simulink model "dragEffects"  (R2016b)
settings: Solver=ode113  StartTime=0.0  StopTime=.5*86400  MaxStep=60  RelTol=1e-6  AbsTol=1e-9
values from neighbouring files (symbols this model uses):
  i = .7854    (= 0.7854)    [PS8.m]
  rINT = [6613.137; 0; 0]    [PS8.m]
  vINT = [0; 7.763631; 0]    [PS8.m]
undefined symbols (not defined in the file or in its folder): AoP, RAAN
settings Model: Creator=rushalrege  LastModifiedBy=rushalrege

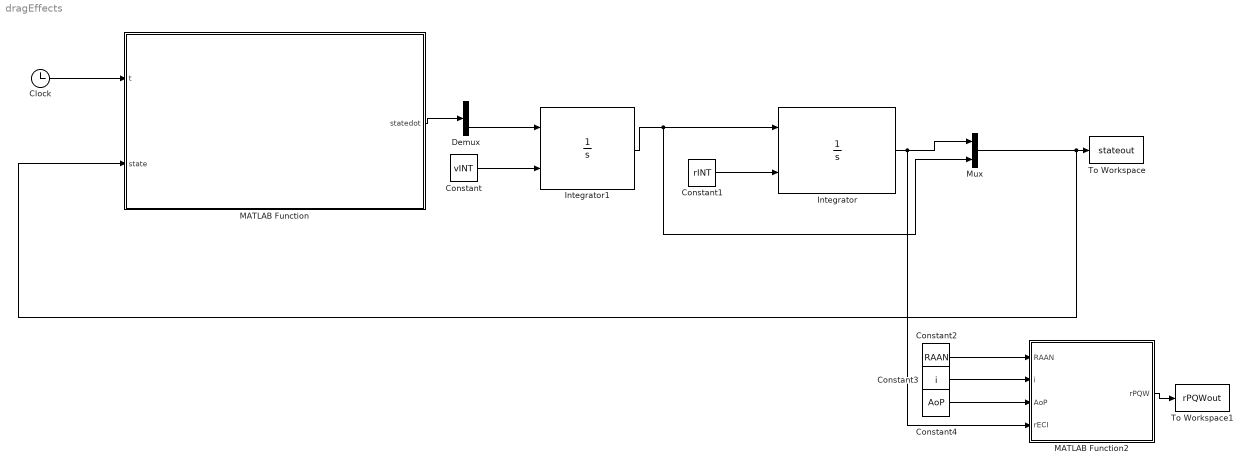
== system dragEffects ==
  Clock : Clock
  Constant : Constant  Value=vINT
  Constant1 : Constant  Value=rINT
  Constant2 : Constant  Value=RAAN
  Constant3 : Constant  Value=i
  Constant4 : Constant  Value=AoP
  Demux : Demux  Outputs=2
  Integrator : Integrator  InitialConditionSource=external
  Integrator1 : Integrator  InitialConditionSource=external
  MATLAB Function : MATLAB Function  TreatAsAtomicUnit=on
  MATLAB Function2 : MATLAB Function  TreatAsAtomicUnit=on
  Mux : Mux  Inputs=2
  To Workspace : ToWorkspace  VariableName=stateout  SampleTime=-1
  To Workspace1 : ToWorkspace  VariableName=rPQWout  SampleTime=-1
  wires:
  Integrator1/1 -> Mux/2, Integrator/1
  Constant/1 -> Integrator1/2
  Constant1/1 -> Integrator/2
  Clock/1 -> MATLAB Function/1(t)
  MATLAB Function/1(statedot) -> Demux/1
  Demux/2 -> Integrator1/1
  Mux/1 -> To Workspace/1, MATLAB Function/2(state)
  Integrator/1 -> MATLAB Function2/4(rECI), Mux/1
  Constant4/1 -> MATLAB Function2/3(AoP)
  Constant3/1 -> MATLAB Function2/2(i)
  Constant2/1 -> MATLAB Function2/1(RAAN)
  MATLAB Function2/1(rPQW) -> To Workspace1/1

== matlab function dragEffects/MATLAB Function ==
  data: t input; statedot output; state input
function statedot = timederivdrag(t,state)

statedot = zeros(6,1);
statedot(1:3) = state(4:6);


statedot(4:6) = (3.986E5 .* -state(1:3)) / norm(state(1:3))^3;

Cd = 2.3;
M = 1500;
A = 2E-5;

h = norm(state(1:3));
p0 = 1.225E9;
H = 10;
h0 = 6378.137;

p = p0 * exp(-((h - h0) / H));
B = Cd * A / M;
vrel = state(4:6) - cross([0; 0; 2*pi/86400],state(1:3));

fdrag = -0.5 .* B .* p .* norm(vrel)^2 .* (vrel / norm(vrel));

statedot(4:6) = statedot(4:6) + fdrag;

end

== matlab function dragEffects/MATLAB Function2 ==
  data: RAAN input; rPQW output; i input; AoP input; rECI input
function rPQW = rIJK2rPQW(RAAN, i, AoP, rECI)

ROM = [cos(-RAAN), sin(-RAAN), 0; -sin(-RAAN), cos(-RAAN), 0; 0, 0, 1];
Ri = [1, 0, 0; 0, cos(-i), sin(-i); 0, -sin(-i), cos(-i)];
Rom = [cos(-AoP), sin(-AoP), 0; -sin(-AoP), cos(-AoP), 0; 0, 0, 1];

R = ROM*Ri*Rom;
R = transpose(R);

rPQW = R*rECI;

end
